simulink model "DiabetesProject"  (R2016a)
settings: Solver=FixedStepAuto  StartTime=0.0  StopTime=48*60  FixedStep=1  RelTol=1e-3
values from neighbouring files (symbols this model uses):
  break_amt = 25/10*(1+mealsize_uncertainty)    (= 2.5)    [DiabetesVariables.m]
  break_timing = 0    [DiabetesVariables.m]
  Cdenc = double(coeffs(Cden))    [Qdesign.m]
  Cnumc = double(coeffs(Cnum))    [Qdesign.m]
  denc = double(coeffs(den))    [Qdesign.m]
  dinner_amt = 60/20*(1+mealsize_uncertainty)    (= 3)    [DiabetesVariables.m]
  dinner_timing = 0    [DiabetesVariables.m]
  idenc = double(coeffs(iden))    [Qdesign.m]
  inumc = [0 double(coeffs(inum))]    [Qdesign.m]
  Ki = -0.075*(1+Ki_uncertainty)    (= -0.075)    [DiabetesVariables.m]
  Ki0 = -0.075    [Qdesign.m]
  Km = 4    [DiabetesVariables.m]
  lunch_amt = 40/15*(1+mealsize_uncertainty)    (= 2.66666666667)    [DiabetesVariables.m]
  lunch_timing = 0    [DiabetesVariables.m]
  numc = [0 double(coeffs(num))]    [Qdesign.m]
  Tdi = 25    [DiabetesVariables.m]
  Tdm = 15    [DiabetesVariables.m]
  Ti = 140    [DiabetesVariables.m]
  Tm = 50    [DiabetesVariables.m]
settings Model: Creator=benma  LastModifiedBy=benma

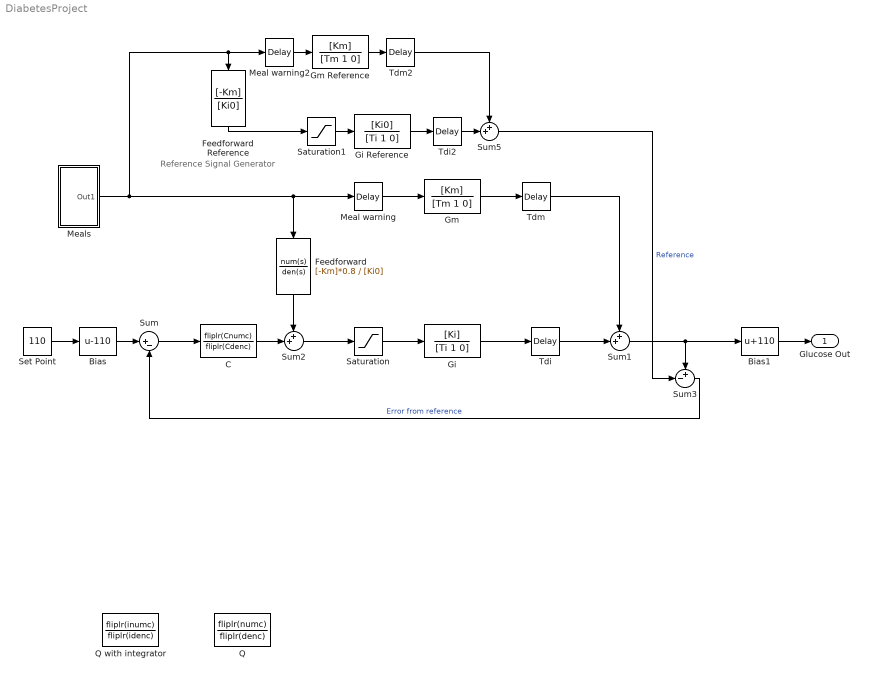
== system DiabetesProject ==
  note: Reference Signal Generator
  Bias : Bias  Bias=-110
  Bias1 : Bias  Bias=110
  C : TransferFcn  Numerator=fliplr(Cnumc)  Denominator=fliplr(Cdenc)
  Feedforward : TransferFcn  Numerator=[-Km]*0.8  Denominator=[Ki0]
  Feedforward Reference : TransferFcn  Numerator=[-Km]  Denominator=[Ki0]
  Gi : TransferFcn  Numerator=[Ki]  Denominator=[Ti 1 0]
  Gi Reference : TransferFcn  Numerator=[Ki0]  Denominator=[Ti 1 0]
  Gm : TransferFcn  Numerator=[Km]  Denominator=[Tm 1 0]
  Gm Reference : TransferFcn  Numerator=[Km]  Denominator=[Tm 1 0]
  Meal warning : TransportDelay  DelayTime=10
  Meal warning2 : TransportDelay  DelayTime=10
  Meals : Subsystem
  Q : TransferFcn  Numerator=fliplr(numc)  Denominator=fliplr(denc)
  Q with integrator : TransferFcn  Numerator=fliplr(inumc)  Denominator=fliplr(idenc)
  Saturation : Saturate  UpperLimit=166  LowerLimit=0
  Saturation1 : Saturate  UpperLimit=166  LowerLimit=0
  Set Point : Constant  Value=110
  Sum : Sum  Inputs=|+-
  Sum1 : Sum  Inputs=++|
  Sum2 : Sum  Inputs=++|
  Sum3 : Sum  Inputs=+-|
  Sum5 : Sum  Inputs=++|
  Tdi : TransportDelay  DelayTime=Tdi
  Tdi2 : TransportDelay  DelayTime=Tdi
  Tdm : TransportDelay  DelayTime=Tdm
  Tdm2 : TransportDelay  DelayTime=Tdm
  Glucose Out : Outport
  wires:
  Gi/1 -> Tdi/1
  Tdi/1 -> Sum1/2
  Gm/1 -> Tdm/1
  Sum1/1 -> Sum3/1, Bias1/1
  Tdm/1 -> Sum1/1
  Set Point/1 -> Bias/1
  Bias/1 -> Sum/1
  Bias1/1 -> Glucose Out/1
  Sum/1 -> C/1
  Saturation/1 -> Gi/1
  Sum2/1 -> Saturation/1
  Gm Reference/1 -> Tdm2/1
  Meals/1(Out1) -> Meal warning/1, Feedforward/1, Meal warning2/1, Feedforward Reference/1
  Sum3/1 -> Sum/2  "Error from reference"
  Gi Reference/1 -> Tdi2/1
  Tdi2/1 -> Sum5/2
  Tdm2/1 -> Sum5/1
  Saturation1/1 -> Gi Reference/1
  Feedforward Reference/1 -> Saturation1/1
  Meal warning/1 -> Gm/1
  Meal warning2/1 -> Gm Reference/1
  C/1 -> Sum2/2
  Feedforward/1 -> Sum2/1
  Sum5/1 -> Sum3/2  "Reference"

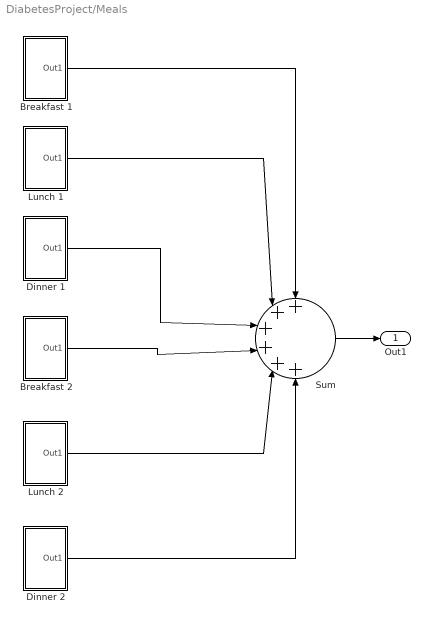
== system DiabetesProject/Meals ==
  Breakfast 1 : Subsystem
  Breakfast 2 : Subsystem
  Dinner 1 : Subsystem
  Dinner 2 : Subsystem
  Lunch 1 : Subsystem
  Lunch 2 : Subsystem
  Sum : Sum  Inputs=++++++
  Out1 : Outport
  wires:
  Breakfast 1/1(Out1) -> Sum/1
  Lunch 1/1(Out1) -> Sum/2
  Dinner 1/1(Out1) -> Sum/3
  Breakfast 2/1(Out1) -> Sum/4
  Lunch 2/1(Out1) -> Sum/5
  Dinner 2/1(Out1) -> Sum/6
  Sum/1 -> Out1/1

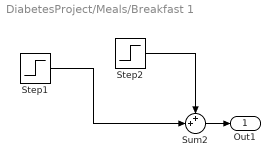
== system DiabetesProject/Meals/Breakfast 1 ==
  Step1 : Step  Time=60+break_timing  After=break_amt  SampleTime=0
  Step2 : Step  Time=70+break_timing  After=-break_amt  SampleTime=0
  Sum2 : Sum  Inputs=++|
  Out1 : Outport
  wires:
  Step2/1 -> Sum2/1
  Sum2/1 -> Out1/1
  Step1/1 -> Sum2/2

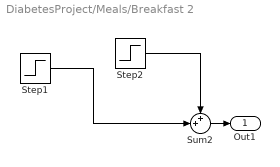
== system DiabetesProject/Meals/Breakfast 2 ==
  Step1 : Step  Time=25*60+break_timing  After=break_amt  SampleTime=0
  Step2 : Step  Time=25*60+10+break_timing  After=-break_amt  SampleTime=0
  Sum2 : Sum  Inputs=++|
  Out1 : Outport
  wires:
  Step2/1 -> Sum2/1
  Sum2/1 -> Out1/1
  Step1/1 -> Sum2/2

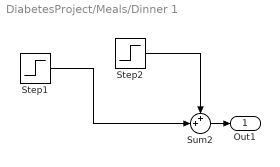
== system DiabetesProject/Meals/Dinner 1 ==
  Step1 : Step  Time=13*60+dinner_timing  After=dinner_amt  SampleTime=0
  Step2 : Step  Time=13*60+20+dinner_timing  After=-dinner_amt  SampleTime=0
  Sum2 : Sum  Inputs=++|
  Out1 : Outport
  wires:
  Step2/1 -> Sum2/1
  Sum2/1 -> Out1/1
  Step1/1 -> Sum2/2

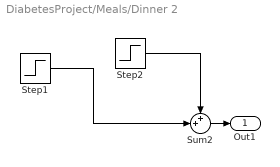
== system DiabetesProject/Meals/Dinner 2 ==
  Step1 : Step  Time=37*60+dinner_timing  After=dinner_amt  SampleTime=0
  Step2 : Step  Time=37*60+20+dinner_timing  After=-dinner_amt  SampleTime=0
  Sum2 : Sum  Inputs=++|
  Out1 : Outport
  wires:
  Step2/1 -> Sum2/1
  Sum2/1 -> Out1/1
  Step1/1 -> Sum2/2

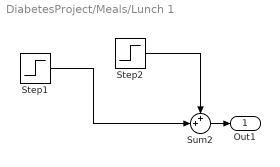
== system DiabetesProject/Meals/Lunch 1 ==
  Step1 : Step  Time=7*60+lunch_timing  After=lunch_amt  SampleTime=0
  Step2 : Step  Time=7*60+15+lunch_timing  After=-lunch_amt  SampleTime=0
  Sum2 : Sum  Inputs=++|
  Out1 : Outport
  wires:
  Step2/1 -> Sum2/1
  Sum2/1 -> Out1/1
  Step1/1 -> Sum2/2

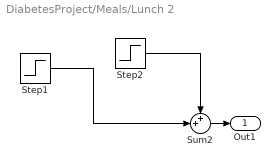
== system DiabetesProject/Meals/Lunch 2 ==
  Step1 : Step  Time=31*60+lunch_timing  After=lunch_amt  SampleTime=0
  Step2 : Step  Time=31*60+15+lunch_timing  After=-lunch_amt  SampleTime=0
  Sum2 : Sum  Inputs=++|
  Out1 : Outport
  wires:
  Step2/1 -> Sum2/1
  Sum2/1 -> Out1/1
  Step1/1 -> Sum2/2
